simulink model "untitled"  (R2020b)
settings: Solver=VariableStepAuto  StartTime=0.0  StopTime=10.0  RelTol=1e-3
libraries: vrlib x3
settings Model: Creator=loren  LastModifiedBy=loren

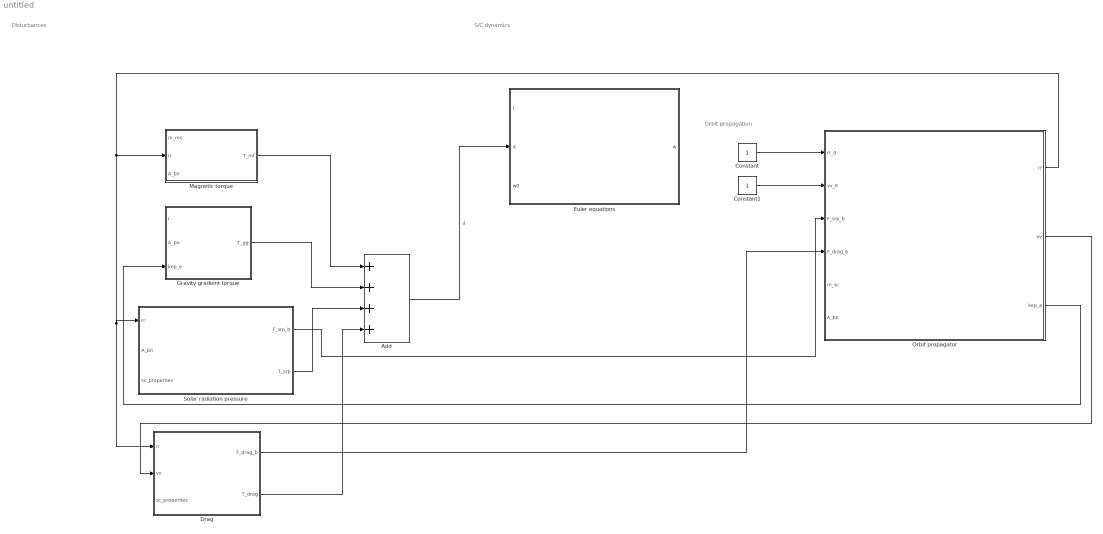
== system untitled ==
  note: S/C dynamics
  note: Orbit propagation
  note: Disturbances
  Add : Sum  Inputs=++++
  Constant : Constant
  Constant1 : Constant
  Drag : Subsystem
  Euler equations : Subsystem
  Gravity gradient torque : Subsystem
  Magnetic torque : Subsystem
  Orbit propagator : Subsystem
  Solar radiation pressure : Subsystem
  wires:
  Magnetic torque/1(T_mf) -> Add/1
  Gravity gradient torque/1(T_gg) -> Add/2
  Solar radiation pressure/2(T_srp) -> Add/3
  Drag/2(T_drag) -> Add/4
  Add/1 -> Euler equations/2(d)  "d"
  Solar radiation pressure/1(F_srp_b) -> Orbit propagator/3(F_srp_b)
  Drag/1(F_drag_b) -> Orbit propagator/4(F_drag_b)
  Constant/1 -> Orbit propagator/1(rr_0)
  Constant1/1 -> Orbit propagator/2(vv_0)
  Orbit propagator/1(rr) -> Drag/1(rr), Solar radiation pressure/1(rr), Magnetic torque/2(rr)
  Orbit propagator/2(vv) -> Drag/2(vv)
  Orbit propagator/3(kep_e) -> Gravity gradient torque/3(kep_e)

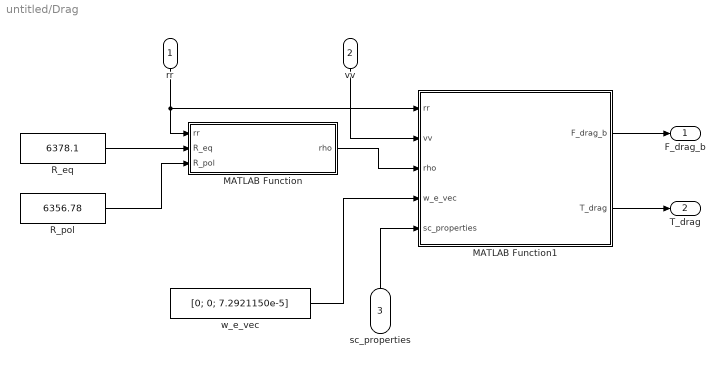
== system untitled/Drag ==
  rr : Inport
  vv : Inport  Port=2
  sc_properties : Inport  Port=3
  MATLAB Function : MATLAB Function  TreatAsAtomicUnit=on
  MATLAB Function1 : MATLAB Function  TreatAsAtomicUnit=on
  R_eq : Constant  Value=6378.1
  R_pol : Constant  Value=6356.78
  w_e_vec : Constant  Value=[0; 0; 7.2921150e-5]
  F_drag_b : Outport
  T_drag : Outport  Port=2
  wires:
  rr/1 -> MATLAB Function1/1(rr), MATLAB Function/1(rr)
  R_eq/1 -> MATLAB Function/2(R_eq)
  R_pol/1 -> MATLAB Function/3(R_pol)
  MATLAB Function/1(rho) -> MATLAB Function1/3(rho)
  sc_properties/1 -> MATLAB Function1/5(sc_properties)
  w_e_vec/1 -> MATLAB Function1/4(w_e_vec)
  MATLAB Function1/1(F_drag_b) -> F_drag_b/1
  MATLAB Function1/2(T_drag) -> T_drag/1
  vv/1 -> MATLAB Function1/2(vv)

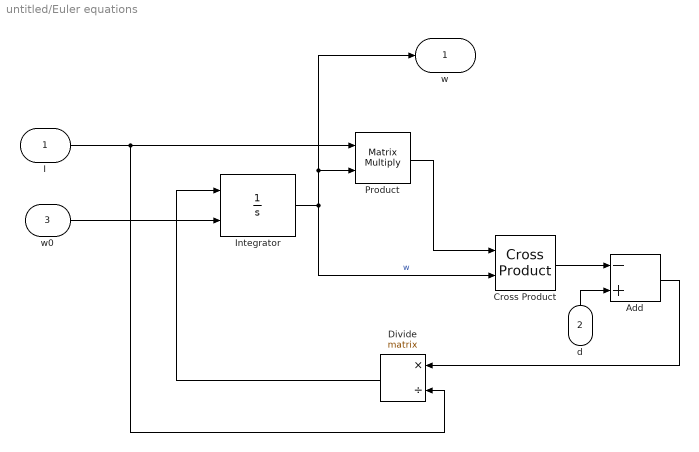
== system untitled/Euler equations ==
  I : Inport
  d : Inport  Port=2
  w0 : Inport  Port=3
  Add : Sum  Inputs=-+
  Cross Product : vrlib/Utilities/Cross Product
  Divide : Product  Inputs=*/  Multiplication=Matrix(*)
  Integrator : Integrator  InitialConditionSource=external
  Product : Product  Multiplication=Matrix(*)
  w : Outport
  wires:
  I/1 -> Divide/2, Product/1
  w0/1 -> Integrator/2
  Integrator/1 -> Product/2, w/1, Cross Product/2  "w"
  Product/1 -> Cross Product/1
  d/1 -> Add/2
  Cross Product/1 -> Add/1
  Add/1 -> Divide/1
  Divide/1 -> Integrator/1

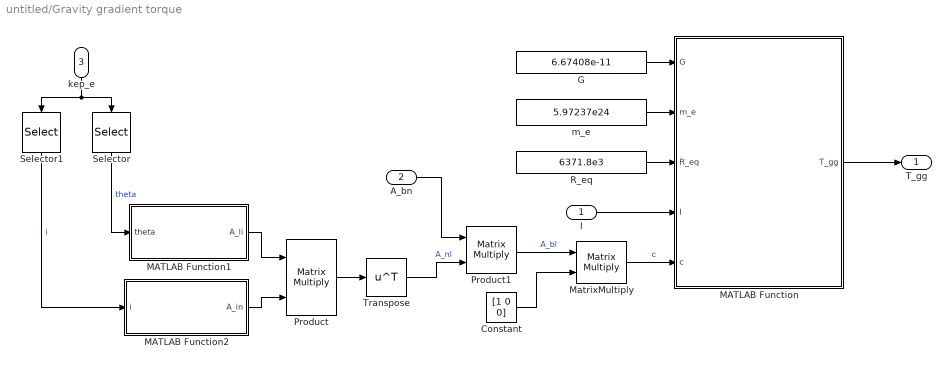
== system untitled/Gravity gradient torque ==
  I : Inport
  A_bn : Inport  Port=2
  kep_e : Inport  Port=3
  Constant : Constant  Value=[1 0 0]
  G : Constant  Value=6.67408e-11
  MATLAB Function : MATLAB Function  TreatAsAtomicUnit=on
  MATLAB Function1 : MATLAB Function  TreatAsAtomicUnit=on
  MATLAB Function2 : MATLAB Function  TreatAsAtomicUnit=on
  MatrixMultiply : Product  Multiplication=Matrix(*)
  Product : Product  Multiplication=Matrix(*)
  Product1 : Product  Multiplication=Matrix(*)
  R_eq : Constant  Value=6371.8e3
  Selector : Selector  InputPortWidth=6  IndexOptions=Index vector (dialog)  Indices=6  OutputSizes=1
  Selector1 : Selector  InputPortWidth=6  IndexOptions=Index vector (dialog)  Indices=3  OutputSizes=1
  Transpose : Math  Operator=transpose  SaturateOnIntegerOverflow=on
  m_e : Constant  Value=5.97237e24
  T_gg : Outport
  wires:
  I/1 -> MATLAB Function/4(I)
  R_eq/1 -> MATLAB Function/3(R_eq)
  G/1 -> MATLAB Function/1(G)
  m_e/1 -> MATLAB Function/2(m_e)
  Product/1 -> Transpose/1
  Transpose/1 -> Product1/2  "A_nl"
  Product1/1 -> MatrixMultiply/1  "A_bl"
  A_bn/1 -> Product1/1
  Constant/1 -> MatrixMultiply/2
  MatrixMultiply/1 -> MATLAB Function/5(c)  "c"
  MATLAB Function/1(T_gg) -> T_gg/1
  kep_e/1 -> Selector/1, Selector1/1
  MATLAB Function2/1(A_in) -> Product/2
  Selector1/1 -> MATLAB Function2/1(i)  "i"
  Selector/1 -> MATLAB Function1/1(theta)  "theta"
  MATLAB Function1/1(A_li) -> Product/1

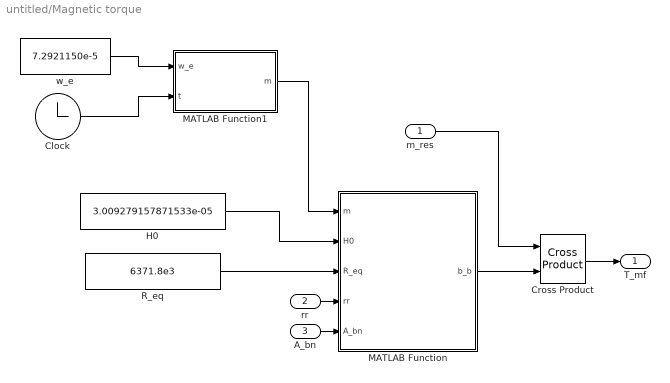
== system untitled/Magnetic torque ==
  m_res : Inport
  rr : Inport  Port=2
  A_bn : Inport  Port=3
  Clock : Clock
  Cross Product : vrlib/Utilities/Cross Product
  H0 : Constant  Value=3.009279157871533e-05
  MATLAB Function : MATLAB Function  TreatAsAtomicUnit=on
  MATLAB Function1 : MATLAB Function  TreatAsAtomicUnit=on
  R_eq : Constant  Value=6371.8e3
  w_e : Constant  Value=7.2921150e-5
  T_mf : Outport
  wires:
  Cross Product/1 -> T_mf/1
  Clock/1 -> MATLAB Function1/2(t)
  m_res/1 -> Cross Product/1
  MATLAB Function/1(b_b) -> Cross Product/2
  H0/1 -> MATLAB Function/2(H0)
  R_eq/1 -> MATLAB Function/3(R_eq)
  w_e/1 -> MATLAB Function1/1(w_e)
  rr/1 -> MATLAB Function/4(rr)
  A_bn/1 -> MATLAB Function/5(A_bn)
  MATLAB Function1/1(m) -> MATLAB Function/1(m)

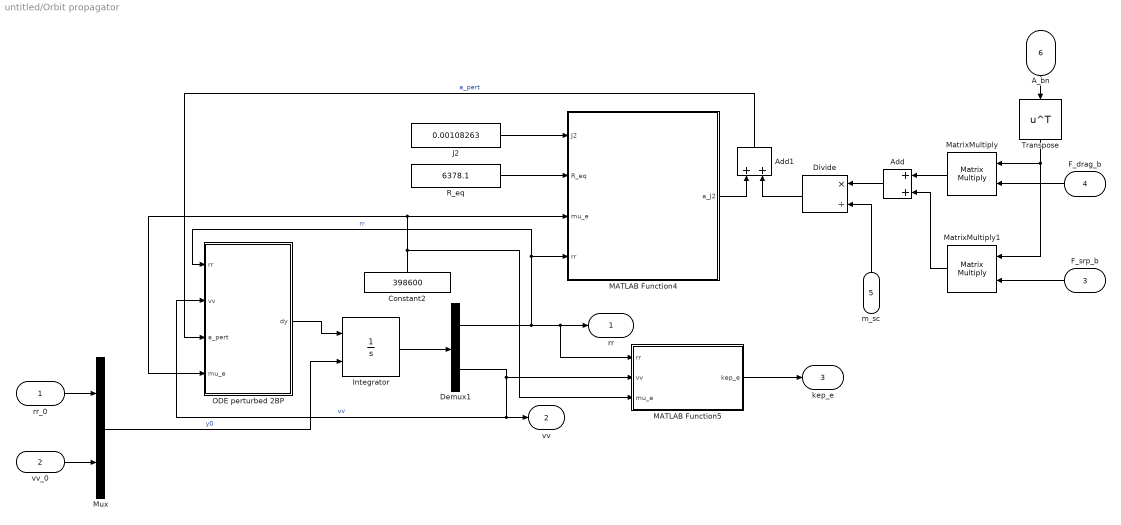
== system untitled/Orbit propagator ==
  rr_0 : Inport
  vv_0 : Inport  Port=2
  F_srp_b : Inport  Port=3
  F_drag_b : Inport  Port=4
  m_sc : Inport  Port=5
  A_bn : Inport  Port=6
  Add : Sum
  Add1 : Sum
  Constant2 : Constant  Value=398600
  Demux1 : Demux  Outputs=[3,3]
  Divide : Product  Inputs=*/
  Integrator : Integrator  InitialConditionSource=external
  J2 : Constant  Value=0.00108263
  MATLAB Function4 : MATLAB Function  TreatAsAtomicUnit=on
  MATLAB Function5 : MATLAB Function  TreatAsAtomicUnit=on
  MatrixMultiply : Product  Multiplication=Matrix(*)
  MatrixMultiply1 : Product  Multiplication=Matrix(*)
  Mux : Mux  Inputs=[3,3]
  ODE perturbed 2BP : Subsystem
  R_eq : Constant  Value=6378.1
  Transpose : Math  Operator=transpose  SaturateOnIntegerOverflow=on
  rr : Outport
  vv : Outport  Port=2
  kep_e : Outport  Port=3
  wires:
  J2/1 -> MATLAB Function4/1(J2)
  R_eq/1 -> MATLAB Function4/2(R_eq)
  Constant2/1 -> MATLAB Function5/3(mu_e), ODE perturbed 2BP/4(mu_e), MATLAB Function4/3(mu_e)
  Integrator/1 -> Demux1/1
  Demux1/1 -> MATLAB Function5/1(rr), rr/1, ODE perturbed 2BP/1(rr), MATLAB Function4/4(rr)  "rr"
  rr_0/1 -> Mux/1
  vv_0/1 -> Mux/2
  ODE perturbed 2BP/1(dy) -> Integrator/1
  Demux1/2 -> vv/1, ODE perturbed 2BP/2(vv), MATLAB Function5/2(vv)  "vv"
  Mux/1 -> Integrator/2  "y0"
  Add1/1 -> ODE perturbed 2BP/3(a_pert)  "a_pert"
  MATLAB Function4/1(a_J2) -> Add1/1
  F_srp_b/1 -> MatrixMultiply1/2
  F_drag_b/1 -> MatrixMultiply/2
  Add/1 -> Divide/1
  m_sc/1 -> Divide/2
  Divide/1 -> Add1/2
  MATLAB Function5/1(kep_e) -> kep_e/1
  A_bn/1 -> Transpose/1
  Transpose/1 -> MatrixMultiply/1, MatrixMultiply1/1
  MatrixMultiply/1 -> Add/1
  MatrixMultiply1/1 -> Add/2

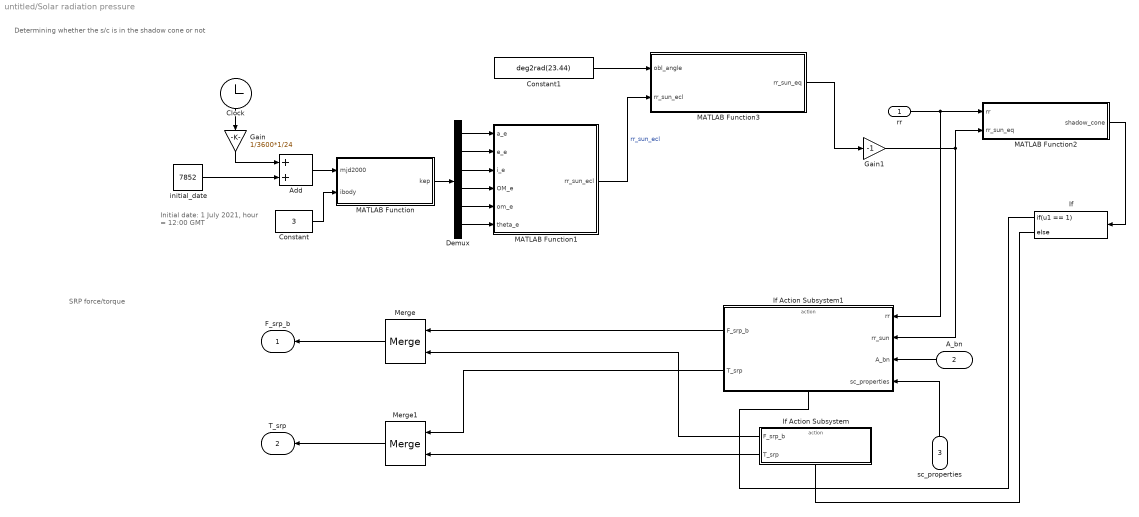
== system untitled/Solar radiation pressure ==
  note: SRP force/torque
  note: Initial date: 1 July 2021,
      | hour = 12:00 GMT
  note: Determining whether the s/c is in the shadow cone or not
  rr : Inport
  A_bn : Inport  Port=2
  sc_properties : Inport  Port=3
  Add : Sum
  Clock : Clock
  Constant : Constant  Value=3
  Constant1 : Constant  Value=deg2rad(23.44)
  Demux : Demux  Outputs=6
  Gain : Gain  Gain=1/3600*1/24
  Gain1 : Gain  Gain=-1
  If : If  IfExpression=u1 == 1
  If Action Subsystem : Subsystem  TreatAsAtomicUnit=on
  If Action Subsystem1 : Subsystem  TreatAsAtomicUnit=on
  MATLAB Function : MATLAB Function  TreatAsAtomicUnit=on
  MATLAB Function1 : MATLAB Function  TreatAsAtomicUnit=on
  MATLAB Function2 : MATLAB Function  TreatAsAtomicUnit=on
  MATLAB Function3 : MATLAB Function  TreatAsAtomicUnit=on
  Merge : Merge
  Merge1 : Merge
  initial_date : Constant  Value=7852
  F_srp_b : Outport
  T_srp : Outport  Port=2
  wires:
  initial_date/1 -> Add/2
  Clock/1 -> Gain/1
  Constant1/1 -> MATLAB Function3/1(obl_angle)
  Add/1 -> MATLAB Function/1(mjd2000)
  Constant/1 -> MATLAB Function/2(ibody)
  Demux/5 -> MATLAB Function1/5(om_e)
  Gain/1 -> Add/1
  Demux/4 -> MATLAB Function1/4(OM_e)
  MATLAB Function3/1(rr_sun_eq) -> Gain1/1
  Demux/6 -> MATLAB Function1/6(theta_e)
  Demux/2 -> MATLAB Function1/2(e_e)
  MATLAB Function1/1(rr_sun_ecl) -> MATLAB Function3/2(rr_sun_ecl)  "rr_sun_ecl"
  MATLAB Function/1(kep) -> Demux/1
  Gain1/1 -> If Action Subsystem1/2(rr_sun), MATLAB Function2/2(rr_sun_eq)
  MATLAB Function2/1(shadow_cone) -> If/1
  Demux/1 -> MATLAB Function1/1(a_e)
  Demux/3 -> MATLAB Function1/3(i_e)
  If/2 -> If Action Subsystem/Action
  If/1 -> If Action Subsystem1/Action
  If Action Subsystem/1(F_srp_b) -> Merge/2
  If Action Subsystem/2(T_srp) -> Merge1/2
  rr/1 -> MATLAB Function2/1(rr), If Action Subsystem1/1(rr)
  Merge/1 -> F_srp_b/1
  Merge1/1 -> T_srp/1
  If Action Subsystem1/1(F_srp_b) -> Merge/1
  If Action Subsystem1/2(T_srp) -> Merge1/1
  A_bn/1 -> If Action Subsystem1/3(A_bn)
  sc_properties/1 -> If Action Subsystem1/4(sc_properties)

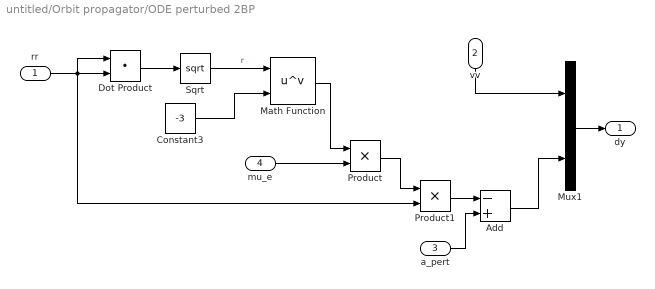
== system untitled/Orbit propagator/ODE perturbed 2BP ==
  rr : Inport
  vv : Inport  Port=2
  a_pert : Inport  Port=3
  mu_e : Inport  Port=4
  Add : Sum  Inputs=-+
  Constant3 : Constant  Value=-3
  Dot Product : DotProduct  InputSameDT=on  OutDataTypeStr=Inherit: Inherit via internal rule
  Math Function : Math  Operator=pow  SaturateOnIntegerOverflow=on
  Mux1 : Mux  Inputs=[3,3]
  Product : Product
  Product1 : Product
  Sqrt : Sqrt  SaturateOnIntegerOverflow=on
  dy : Outport
  wires:
  rr/1 -> Dot Product/1, Product1/2, Dot Product/2
  Add/1 -> Mux1/2
  Math Function/1 -> Product/1
  Mux1/1 -> dy/1
  Dot Product/1 -> Sqrt/1
  Product1/1 -> Add/1
  Product/1 -> Product1/1
  Constant3/1 -> Math Function/2
  a_pert/1 -> Add/2
  Sqrt/1 -> Math Function/1  "r"
  vv/1 -> Mux1/1
  mu_e/1 -> Product/2

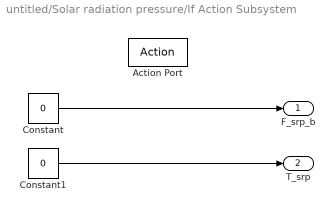
== system untitled/Solar radiation pressure/If Action Subsystem ==
  Action Port : ActionPort  ActionPortLabel=else
  Constant : Constant  Value=0
  Constant1 : Constant  Value=0
  F_srp_b : Outport
  T_srp : Outport  Port=2
  wires:
  Constant/1 -> F_srp_b/1
  Constant1/1 -> T_srp/1

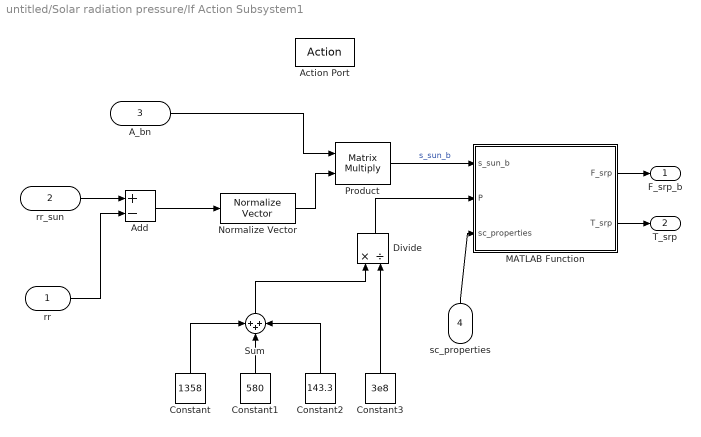
== system untitled/Solar radiation pressure/If Action Subsystem1 ==
  rr : Inport
  rr_sun : Inport  Port=2
  A_bn : Inport  Port=3
  sc_properties : Inport  Port=4
  Action Port : ActionPort  ActionPortLabel=if(u1 == 1)
  Add : Sum  Inputs=+-
  Constant : Constant  Value=1358
  Constant1 : Constant  Value=580
  Constant2 : Constant  Value=143.3
  Constant3 : Constant  Value=3e8
  Divide : Product  Inputs=*/
  MATLAB Function : MATLAB Function  TreatAsAtomicUnit=on
  Normalize Vector : vrlib/Utilities/Normalize Vector  maxzero=0
  Product : Product  Multiplication=Matrix(*)
  Sum : Sum  Inputs=+++
  F_srp_b : Outport
  T_srp : Outport  Port=2
  wires:
  A_bn/1 -> Product/1
  rr_sun/1 -> Add/1
  Product/1 -> MATLAB Function/1(s_sun_b)  "s_sun_b"
  Normalize Vector/1 -> Product/2
  Add/1 -> Normalize Vector/1
  MATLAB Function/1(F_srp) -> F_srp_b/1
  MATLAB Function/2(T_srp) -> T_srp/1
  sc_properties/1 -> MATLAB Function/3(sc_properties)
  Constant1/1 -> Sum/2
  Constant2/1 -> Sum/3
  Constant/1 -> Sum/1
  Sum/1 -> Divide/1
  Constant3/1 -> Divide/2
  Divide/1 -> MATLAB Function/2(P)
  rr/1 -> Add/2

== matlab function untitled/Gravity gradient torque/MATLAB Function1 ==
  data: theta input; A_li output
function A_li = inclined_to_orbital(theta)

A_li = [cos(theta), sin(theta), 0;...
    -sin(theta), cos(theta), 0;...
    0, 0, 1];

end

== matlab function untitled/Gravity gradient torque/MATLAB Function2 ==
  data: i input; A_in output
function A_in = inertial_to_inclined(i)

A_in = [1, 0, 0;...
    0, cos(i), sin(i);...
    0, -sin(i), cos(i)];

end

== matlab function untitled/Drag/MATLAB Function ==
  data: rr input; rho output; R_eq input; R_pol input
function rho = CIRA72_density(rr, R_eq, R_pol)
% 
% Function to compute the atmosphere density using the CIRA-72 model.
% 
% INPUT:
%  rr   [3,1]       Position Vector
%  R_eq  [1]        Equatorial radius of the Earth
%  R_pol [1]        Polar radius of the Earth
%
% OUTPUT:
%   rho             Density [kg/m^3]
% 

lat = pi/2 - acos(rr(3)/norm(rr)); % Latitude of the satellite

% Earth's radius for the specified latitude:
a = R_pol*cos(lat);
b = R_eq*sin(lat);
R = sqrt((R_eq^2*R_pol^2)/(a^2+b^2));

alt = norm(rr) - R; % Local altitude of the satellite

if alt<=180
    h0 = 150;
    rho0 = 2.070*1e-9;
    H = 22.523;
elseif alt<=200 && alt>180
    h0 = 180;
    rho0 = 5.464*1e-10;
    H = 29.740;
elseif alt<=250 && alt>200
    h0 = 200;
    rho0 = 2.789*1e-10;
    H = 37.105;
elseif alt<=300 && alt>250
    h0 = 250;
    rho0 = 7.248*1e-11;
    H = 45.546;  
elseif alt<=350 && alt>300
    h0 = 300;
    rho0 = 2.418*1e-11;
    H = 53.628;
elseif alt<=400 && alt>350
    h0 = 350;
    rho0 = 9.158*1e-12;
    H = 53.298;
elseif alt<=450 && alt>400
    h0 = 400;
    rho0 = 3.725*1e-12;
    H = 58.515;
elseif alt<=500 && alt>450
    h0 = 450;
    rho0 = 1.585*1e-12;
    H = 60.828;
end

rho = rho0*exp(-(alt-h0)/H);

end

== matlab function untitled/Drag/MATLAB Function1 ==
  data: rr input; vv input; rho input; F_drag_b output; w_e_vec input; sc_properties input; T_drag output
function [F_drag_b, T_drag] = drag(rr, vv, rho, w_e_vec, sc_properties)

v_atm = cross(we,rr*1e3); % [m/s]
v_rel = vv*1e3 - v_atm; % [m/s]

end

== matlab function untitled/Magnetic torque/MATLAB Function1 ==
  data: w_e input; m output; t input
function m = m_vector(w_e, t)

m = [sind(11.5)*cos(w_e*t),...
    sind(11.5)*sin(w_e*t),...
    cosd(11.5)];

end

== matlab function untitled/Magnetic torque/MATLAB Function ==
  data: m input; H0 input; R_eq input; rr input; b_b output; A_bn input
function b_b = magnetic_dipole(m, H0, R_eq, rr, A_bn)

r_norm = norm(rr);
r_vec = rr/norm(rr)*1e3;

b_n = R_eq^3*H0/(r_norm^3)*(3*dot(m,r_vec)*r_vec - m);

b_b = A_bn*b_n;

end

== matlab function untitled/Gravity gradient torque/MATLAB Function ==
  data: G input; T_gg output; m_e input; R_eq input; I input; c input
function T_gg = gravity_gradient(G, m_e, R_eq, I, c)

c1 = c(1);
c2 = c(2);
c3 = c(3);
Ix = I(1,1);
Iy = I(2,2);
Iz = I(3,3);

T_gg = 3*G*m_e/(R_eq^3)*[(Iz - Iy)*c2*c3,...
    (Ix - Iz)*c1*c3,...
    (Iy - Ix)*c1*c2];

end

== matlab function untitled/Solar radiation pressure/MATLAB Function ==
  data: mjd2000 input; kep output; ibody input
function  kep = uplanet(mjd2000, ibody)

% uplanet.m - Analytical ephemerides for planets
%
% PROTOTYPE:
%  [kep, ksun] = uplanet (mjd2000, ibody);
%
% DESCRIPTION:
%   Planetary orbital elements are restituited in a Sun-centred ecliptic 
%   system.
%   These ephemerides were succesfully compared with JPL/NAIF/SPICE
%   ephemerides using de405.bps.
%
%  INPUT :
%	mjd2000[1]  Time, modified Julian day since 01/01/2000, 12:00 noon
%               (MJD2000 = MJD-51544.5)
%	ibody[1]    Integer number identifying the celestial body (< 11)
%                   1:   Mercury
%                   2:   Venus
%                   3:   Earth
%                   4:   Mars
%                   5:   Jupiter
%                   6:   Saturn
%                   7:   Uranus
%                   8:   Neptune
%                   9:   Pluto
%                   10:  Sun
%
%  OUTPUT:
%	kep[6]    	Mean Keplerian elements of date
%                 kep = [a e i Om om theta] [km, rad]
%	ksun[1]     Gravity constant of the Sun [km^3/s^2]
%
%   Note: The ephemerides of the Moon are given by EphSS_kep, according to
%           to the algorithm in ephMoon.m
%
%  FUNCTIONS CALLED:
%   (none)
%
% AUTHOR:
%   P. Dysli, 1977
%
% PREVIOUS VERSION:
%   P. Dysli, 1977, MATLAB, uplanet.m
%       - Header and function name in accordance with guidlines.
%
%  CHANGELOG:
%   28/12/06, Camilla Colombo: tidied up
%   10/01/2007, REVISION, Matteo Ceriotti 
%   03/05/2008, Camilla Colombo: Case 11 deleted.
%   11/09/2008, Matteo Ceriotti, Camilla Colombo:
%       - All ephemerides shifted 0.5 days back in time. Now mjd2000 used
%           in this function is referred to 01/01/2000 12:00. In the old
%           version it was referred to 02/01/2000 00:00.
%       - Corrected ephemeris of Pluto.
%   04/10/2010, Camilla Colombo: Header and function name in accordance
%       with guidlines.
%
% -------------------------------------------------------------------------

DEG2RAD=pi/180;

G=6.67259e-20;
msun=1.988919445342813e+030;
ksun=msun*G;

KM  = 149597870.66;

%  T = JULIAN CENTURIES SINCE 31/12/1899 at 12:00
T   = (mjd2000 + 36525)/36525.00;
TT  = T*T;
TTT = T*TT;
kep(1)=T*0;

%
%  CLASSICAL PLANETARY ELEMENTS ESTIMATION IN MEAN ECLIPTIC OF DATE
%
switch round(ibody)
    
    %
    %  MERCURY
    %
    case 1
        kep(1) = 0.38709860;
        kep(2) = 0.205614210 + 0.000020460*T - 0.000000030*TT;
        kep(3) = 7.002880555555555560 + 1.86083333333333333e-3*T - 1.83333333333333333e-5*TT;
        kep(4) = 4.71459444444444444e+1 + 1.185208333333333330*T + 1.73888888888888889e-4*TT;
        kep(5) = 2.87537527777777778e+1 + 3.70280555555555556e-1*T +1.20833333333333333e-4*TT;
        XM   = 1.49472515288888889e+5 + 6.38888888888888889e-6*T;
        kep(6) = 1.02279380555555556e2 + XM*T;
    %
    %  VENUS
    %
    case 2
        kep(1) = 0.72333160;
        kep(2) = 0.006820690 - 0.000047740*T + 0.0000000910*TT;
        kep(3) = 3.393630555555555560 + 1.00583333333333333e-3*T - 9.72222222222222222e-7*TT;
        kep(4) = 7.57796472222222222e+1 + 8.9985e-1*T + 4.1e-4*TT;
        kep(5) = 5.43841861111111111e+1 + 5.08186111111111111e-1*T -1.38638888888888889e-3*TT;
        XM   = 5.8517803875e+4 + 1.28605555555555556e-3*T;
        kep(6) = 2.12603219444444444e2 + XM*T;
    %
    %  EARTH
    %
    case 3
        kep(1) = 1.000000230;
        kep(2) = 0.016751040 - 0.000041800*T - 0.0000001260*TT;
        kep(3) = 0.00;
    	kep(4) = 0.00;
      	kep(5) = 1.01220833333333333e+2 + 1.7191750*T + 4.52777777777777778e-4*TT + 3.33333333333333333e-6*TTT;
     	XM   = 3.599904975e+4 - 1.50277777777777778e-4*T - 3.33333333333333333e-6*TT;
     	kep(6) = 3.58475844444444444e2 + XM*T;
    %
    %  MARS
    %
    case 4
        kep(1) = 1.5236883990;
        kep(2) = 0.093312900 + 0.0000920640*T - 0.0000000770*TT;
        kep(3) = 1.850333333333333330 - 6.75e-4*T + 1.26111111111111111e-5*TT;
        kep(4) = 4.87864416666666667e+1 + 7.70991666666666667e-1*T - 1.38888888888888889e-6*TT - 5.33333333333333333e-6*TTT;
        kep(5) = 2.85431761111111111e+2 + 1.069766666666666670*T +  1.3125e-4*TT + 4.13888888888888889e-6*TTT;
        XM   = 1.91398585e+4 + 1.80805555555555556e-4*T + 1.19444444444444444e-6*TT;
        kep(6) = 3.19529425e2 + XM*T;
    %
    %  JUPITER
    %
    case 5
        kep(1) = 5.2025610;
        kep(2) = 0.048334750 + 0.000164180*T  - 0.00000046760*TT -0.00000000170*TTT;
        kep(3) = 1.308736111111111110 - 5.69611111111111111e-3*T +  3.88888888888888889e-6*TT;
        kep(4) = 9.94433861111111111e+1 + 1.010530*T + 3.52222222222222222e-4*TT - 8.51111111111111111e-6*TTT;
        kep(5) = 2.73277541666666667e+2 + 5.99431666666666667e-1*T + 7.0405e-4*TT + 5.07777777777777778e-6*TTT;
        XM   = 3.03469202388888889e+3 - 7.21588888888888889e-4*T + 1.78444444444444444e-6*TT;
        kep(6) = 2.25328327777777778e2 + XM*T;
    %
    %  SATURN
    %
	case 6
        kep(1) = 9.5547470;
        kep(2) = 0.055892320 - 0.00034550*T - 0.0000007280*TT + 0.000000000740*TTT;
        kep(3) = 2.492519444444444440 - 3.91888888888888889e-3*T - 1.54888888888888889e-5*TT + 4.44444444444444444e-8*TTT;
        kep(4) = 1.12790388888888889e+2 + 8.73195138888888889e-1*T -1.52180555555555556e-4*TT - 5.30555555555555556e-6*TTT;
        kep(5) = 3.38307772222222222e+2 + 1.085220694444444440*T + 9.78541666666666667e-4*TT + 9.91666666666666667e-6*TTT;
        XM   = 1.22155146777777778e+3 - 5.01819444444444444e-4*T - 5.19444444444444444e-6*TT;
        kep(6) = 1.75466216666666667e2 + XM*T;
    %
    %  URANUS
    %
    case 7
        kep(1) = 19.218140;
        kep(2) = 0.04634440 - 0.000026580*T + 0.0000000770*TT;
        kep(3) = 7.72463888888888889e-1 + 6.25277777777777778e-4*T + 3.95e-5*TT;
        kep(4) = 7.34770972222222222e+1 + 4.98667777777777778e-1*T + 1.31166666666666667e-3*TT;
        kep(5) = 9.80715527777777778e+1 + 9.85765e-1*T - 1.07447222222222222e-3*TT - 6.05555555555555556e-7*TTT;
        XM   = 4.28379113055555556e+2 + 7.88444444444444444e-5*T + 1.11111111111111111e-9*TT;
        kep(6) = 7.26488194444444444e1 + XM*T;
    %
    %  NEPTUNE
    %
    case 8
        kep(1) = 30.109570;
        kep(2) = 0.008997040 + 0.0000063300*T - 0.0000000020*TT;
        kep(3) = 1.779241666666666670 - 9.54361111111111111e-3*T - 9.11111111111111111e-6*TT;
        kep(4) = 1.30681358333333333e+2 + 1.0989350*T + 2.49866666666666667e-4*TT - 4.71777777777777778e-6*TTT;
        kep(5) = 2.76045966666666667e+2 + 3.25639444444444444e-1*T + 1.4095e-4*TT + 4.11333333333333333e-6*TTT;
        XM   = 2.18461339722222222e+2 - 7.03333333333333333e-5*T;
        kep(6) = 3.77306694444444444e1 + XM*T;
    %
    %  PLUTO
    %
    case 9
        kep(1) = 39.481686778174627;
        kep(2) = 2.4467e-001;
        kep(3) = 17.150918639446061;
        kep(4) = 110.27718682882954;
        kep(5) = 113.77222937912757;
        XM   = 4.5982945101558835e-008;
        kep(6) = 1.5021e+001 + XM*mjd2000*86400;
    %
    %  SUN
    %
    case 10
        kep = [0 0 0 0 0 0];
    %
    %  MOON (AROUND EARTH)
    %
%     case 11
%         msun=59.736e23;
%         ksun=msun*G;
%         kep(1) = 0.0025695549067660;
%         kep(2) = 0.0549004890;
%         kep(3) = 5.145396388888888890;
%         kep(4) = 2.59183275e+2  - 1.93414200833333333e+3*T + 2.07777777777777778e-3*TT + 2.22222222222222222e-6*TTT;
%         kep(4) = mod(kep(4) + 108e3, 360);
%         kep(5) = 7.51462805555555556e+1    + 6.00317604166666667e+3*T - 1.24027777777777778e-2*TT - 1.47222222222222222e-5*TTT;
%         kep(5) = mod(kep(5), 360);
%         XM   = 4.77198849108333333e+5    + 9.19166666666666667e-3*T  + 1.43888888888888889e-5*TT;
%         kep(6) = 2.96104608333333333e2     + XM                    *T;
    
    otherwise
	disp(ibody)
    if round(ibody)==11
        error('no planet in the list. For the Moon use EphSS_kep instead')
    else
        error('no planet in the list')
    end
end
  
%
%  CONVERSION OF AU INTO KM, DEG INTO RAD AND DEFINITION OF  XMU
%
 
kep(1)   = kep(1)*KM;       % a [km]
kep(3:6) = kep(3:6)*DEG2RAD;    % Transform from deg to rad
kep(6)   = mod(kep(6),2*pi);
% XMU  = (XM*DEG2RAD/(864000*365250))^2*kep(1)^3;
phi    = kep(6);          % phi is the eccentric anomaly, uses kep(6)=M as a first guess
     
for i=1:5
    g       = kep(6)-(phi-kep(2)*sin(phi)); 
	g_primo = (-1+kep(2)*cos(phi));
 	phi     = phi-g/g_primo;   % Computes the eccentric anomaly kep
end 

theta=2*atan(sqrt((1+kep(2))/(1-kep(2)))*tan(phi/2));

kep(6)=theta;

return

== matlab function untitled/Solar radiation pressure/MATLAB Function1 ==
  data: a_e input; rr_sun_ecl output; e_e input; i_e input; OM_e input; om_e input; theta_e input
function rr_sun_ecl = kep2car(a_e,e_e,i_e,OM_e,om_e,theta_e)
% 
% Function to compute position and velocity vectors of the satellite the 
% keplerian elements.
% 
% INPUT:
%  a [1]       Semimajor axis [km]
%  e [1]       Eccentricity [-]
%  i [1]       Inclination angle [rad]
%  OM [1]      Right ascention of the ascending node [rad]
%  om [1]      Anomaly of the pericenter [rad]
%  th [1]      True anomaly [rad]
%  MU [1]      Gravitational parameter of the primary [km^3/s^2]
% 
% OUTPUT:
%  rr [3,1]    Position vector in inertial frame [km]
%  vv [3,1]    Velocity vector in inertial frame [km/s]
% 

p = a_e*(1-e_e^2);
r = p/(1+e_e*cos(theta_e));

rr_sun_ecl = r*[cos(th);sin(th);0];

ROM = [ cos(OM_e) sin(OM_e) 0; -sin(OM_e) cos(OM_e) 0; 0 0 1];
Ri = [ 1 0 0; 0 cos(i_e) sin(i_e); 0 -sin(i_e) cos(i_e)];
Rom = [ cos(om_e) sin(om_e) 0; -sin(om_e) cos(om_e) 0; 0 0 1];

T = Rom*Ri*ROM;

rr_sun_ecl = T'*rr_sun_ecl;

end

== matlab function untitled/Solar radiation pressure/MATLAB Function2 ==
  data: rr input; shadow_cone output; rr_sun_eq input
function shadow_cone = cone(rr, rr_sun_eq)

% PROTOTYPE:
%  shadow_cone = cone(rr_sc, rr_sun)
% 
% DESCRIPTION:
%   This function returns a parameter that is 1 if the s/c is out of the 
%   planet's shadow cone (SRP effects considerable) or 0 if the s/c is 
%   inside the planet's shadow cone (NO SRP)
% 
% INPUT:
% rr_sc:            geocentric position vector of the s/c
% rr_sun_eq:        geocentric position vector of the sun
%
% OUTPUT:
% shadow_cone:      boolean parameter (0 or 1)
%
% CONTRIBUTORS:
% Velo Giacomo
%
% VERSIONS:
% 2019-12-10 first version
%
% CALLED FUNCTIONS:
%     none


R_e = 6378.137;
r_sc = norm(rr);     
r_sun = norm(rr_sun_eq);
% Angle between s/c geocentric position and the tangent to Earth's surface
theta_sc = acos(R_e/r_sc);
% Angle between sun geocentric position and the tangent to Earth's surface
theta_sun = acos(R_e/r_sun);
% Angle between s/c geocentric position and sun geocentric position
theta = acos(dot(rr, rr_sun_eq)/(r_sc*r_sun));

% If the s/c is inside the shadow cone of the planet the value of
% shadow_cone will be = 0

    if theta_sc + theta_sun <= theta
        shadow_cone = 0;
    else
        shadow_cone = 1;
    end

end

== matlab function untitled/Solar radiation pressure/MATLAB Function3 ==
  data: obl_angle input; rr_sun_eq output; rr_sun_ecl input
function rr_sun_eq = ecliptic_to_equatorial(obl_angle, rr_sun_ecl)


% Rotation matrix from ecliptic to equatorial
RR_ecl = [1   0   0;
    0  cos(obl_angle)  -sin(obl_angle);
    0  sin(obl_angle)  cos(obl_angle)];

% Planet position in equatorial
rr_sun_eq = RR_ecl * rr_sun_ecl; % Sun-Centered-Ecliptic -> ECI

end

== matlab function untitled/Orbit propagator/MATLAB Function4 ==
  data: J2 input; a_J2 output; R_eq input; mu_e input; rr input
function a_J2 = J2_perturb(J2, R_eq, mu_e, rr)

r = norm(rr);
rx = rr(1);
ry = rr(2);
rz = rr(3);

a_J2 = 3/2*J2*mu_e*R_eq^2/(rr^4)*[rx/r*(5*(rz/r)^2 - 1),...
    ry/r*(5*(rz/r)^2 - 1),...
    rz/r*(5*(rz/r)^2 - 3)];

end

== matlab function untitled/Orbit propagator/MATLAB Function5 ==
  data: rr input; kep_e output; vv input; mu_e input
function kep_e = car2kep(rr, vv, mu_e)

r = norm(rr);
v = norm(vv);

hh = cross(r,v);
h = norm(hh);
i = acos(hh(3)/h);

a = -mu_e/2*1/(v^2/2 - mu_e/r);

k = [0 0 1];
nn = cross(k,h);
nn = nn/norm(nn);

if nn(2) < 0
    OM = 2*pi - acos(nn(1));
else
    OM = acos(nn(1));
end

ee = cross(v,h)/mu_e - rr/r;
e = norm(ee);

if e(3) < 0
    om = 2*pi - acos(dot(nn,ee)/e);
else
    om = acos(dot(nn,ee)/e);
end

vr = dot(rr,vv);

if vr < 0
    theta = 2*pi - acos(dot(rr,ee)/r/e);
else
    theta = acos(dot(rr,ee)/r/e);
end

kep_e = [a, e, i, OM, om, theta];

end

== matlab function untitled/Solar radiation pressure/If Action Subsystem1/MATLAB Function ==
  data: s_sun_b input; P input; F_srp output; sc_properties input; T_srp output
function [F_srp, T_srp] = srp(s_sun_b, P, sc_properties)


end
